simulink model "Simulation"  (R2023a)
settings: Solver=VariableStepAuto  StartTime=0.0  StopTime=5.0  RelTol=1e-3
values from neighbouring files (symbols this model uses):
  Bm = 0.00071*2    (= 0.00142)    [induction_parameter.m]
  J = 0.0038*1.5    (= 0.0057)    [induction_parameter.m]
  Llr = Lls    (= 0.303)    [induction_parameter.m]
  Lls = 4.928-4.625    (= 0.303)    [induction_parameter.m]
  Lm = Lms    (= 4.625)    [induction_parameter.m]
  omega = 0    [induction_parameter.m]
  p = 4    [induction_parameter.m]
  r_r = 40.5    [induction_parameter.m]
  r_s = 79.13    [induction_parameter.m]
  Vm = 310    [induction_parameter.m]
settings Model: Creator=QUDUS  LastModifiedBy=QUDUS

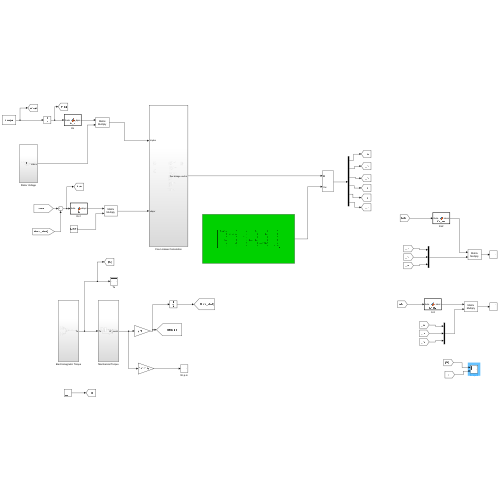
[thumbnail: Simulink's stored preview of the top-level diagram]
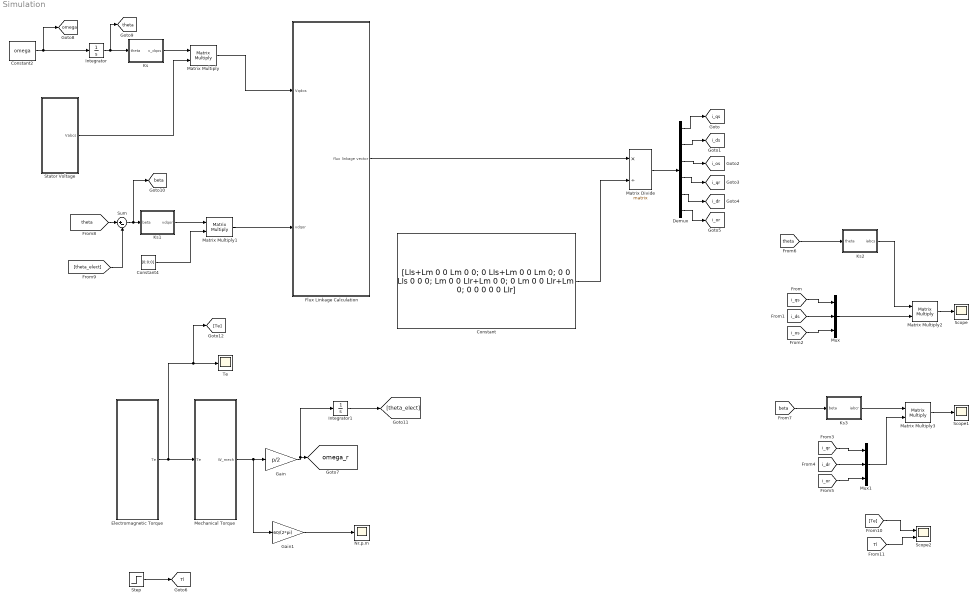
== system Simulation ==
  Constant : Constant  Value=[Lls+Lm 0 0 Lm 0 0; 0 Lls+Lm 0 0 Lm 0; 0 0 Lls 0 0 0; Lm 0 0 Llr+Lm 0 0; 0 Lm 0 0 Llr+Lm 0; 0 0 0 0 0 Llr]
  Constant2 : Constant  Value=omega
  Constant4 : Constant  Value=[0;0;0]
  Demux : Demux  Outputs=6
  Electromagnetic Torque : Subsystem
  Flux Linkage Calculation : Subsystem
  Gain : Gain  Gain=p/2
  Gain1 : Gain  Gain=60/(2*pi)
  Integrator : Integrator
  Integrator1 : Integrator
  Ks : MATLAB Function  TreatAsAtomicUnit=on
  Ks1 : MATLAB Function  TreatAsAtomicUnit=on
  Ks2 : MATLAB Function  TreatAsAtomicUnit=on
  Ks3 : MATLAB Function  TreatAsAtomicUnit=on
  Matrix Divide : Product  Inputs=*/  Multiplication=Matrix(*)
  Matrix Multiply{,1..3} (4 alike) : Product  Multiplication=Matrix(*)
  Mechanical Torque : Subsystem
  Mux : Mux  Inputs=3
  Mux1 : Mux  Inputs=3
  Nr.p.m : Scope
  Scope : Scope
  Scope1 : Scope
  Scope2 : Scope  NumInputPorts=2
  Stator Voltage : Subsystem
  Step : Step  Time=3  After=0.6  SampleTime=0
  Sum : Sum  Inputs=|+-
  Te : Scope
  tag scope: Tl=global, beta=global, i_dr=global, i_ds=global, i_or=global, i_os=global, i_qr=global, i_qs=global, omega=global, omega_r=global, theta=global
  wires:
  Flux Linkage Calculation/1(flux linkage vector) -> Matrix Divide/1
  Constant/1 -> Matrix Divide/2
  Matrix Divide/1 -> Demux/1
  Demux/1 -> [i_qs]
  Demux/2 -> [i_ds]
  Demux/3 -> [i_os]
  Demux/4 -> [i_qr]
  Demux/5 -> [i_dr]
  Demux/6 -> [i_or]
  Step/1 -> [Tl]
  Mechanical Torque/1(W_mech) -> Gain1/1, Gain/1
  Gain1/1 -> Nr.p.m/1
  Gain/1 -> Integrator1/1, [omega_r]
  Ks/1(v_dqos) -> Matrix Multiply/1
  Matrix Multiply/1 -> Flux Linkage Calculation/1(Vqdos)
  Constant2/1 -> Integrator/1, [omega]
  Integrator/1 -> [theta], Ks/1(theta)
  Stator Voltage/1(Vabcs) -> Matrix Multiply/2
  Ks1/1(vdqor) -> Matrix Multiply1/1
  Matrix Multiply1/1 -> Flux Linkage Calculation/2(vdqor)
  Constant4/1 -> Matrix Multiply1/2
  Sum/1 -> [beta], Ks1/1(beta)
  [i_qs] -> Mux/1
  [i_ds] -> Mux/2
  [i_os] -> Mux/3
  Matrix Multiply2/1 -> Scope/1
  [beta] -> Ks3/1(beta)
  Matrix Multiply3/1 -> Scope1/1
  Integrator1/1 -> [theta_elect]
  [theta] -> Sum/1
  [theta_elect] -> Sum/2
  [theta] -> Ks2/1(theta)
  Ks2/1(iabcs) -> Matrix Multiply2/1
  Mux/1 -> Matrix Multiply2/2
  [i_qr] -> Mux1/1
  [i_dr] -> Mux1/2
  [i_or] -> Mux1/3
  Ks3/1(iabcr) -> Matrix Multiply3/1
  Mux1/1 -> Matrix Multiply3/2
  Electromagnetic Torque/1(Te) -> [Te], Te/1, Mechanical Torque/1(Te)
  [Te] -> Scope2/1
  [Tl] -> Scope2/2

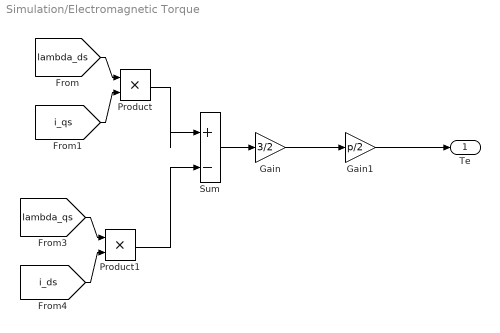
== system Simulation/Electromagnetic Torque ==
  Gain : Gain  Gain=3/2
  Gain1 : Gain  Gain=p/2
  Product : Product
  Product1 : Product
  Sum : Sum  Inputs=|+-
  Te : Outport
  wires:
  Sum/1 -> Gain/1
  Gain/1 -> Gain1/1
  Gain1/1 -> Te/1
  [lambda_ds] -> Product/1
  [i_qs] -> Product/2
  Product/1 -> Sum/1
  [lambda_qs] -> Product1/1
  [i_ds] -> Product1/2
  Product1/1 -> Sum/2

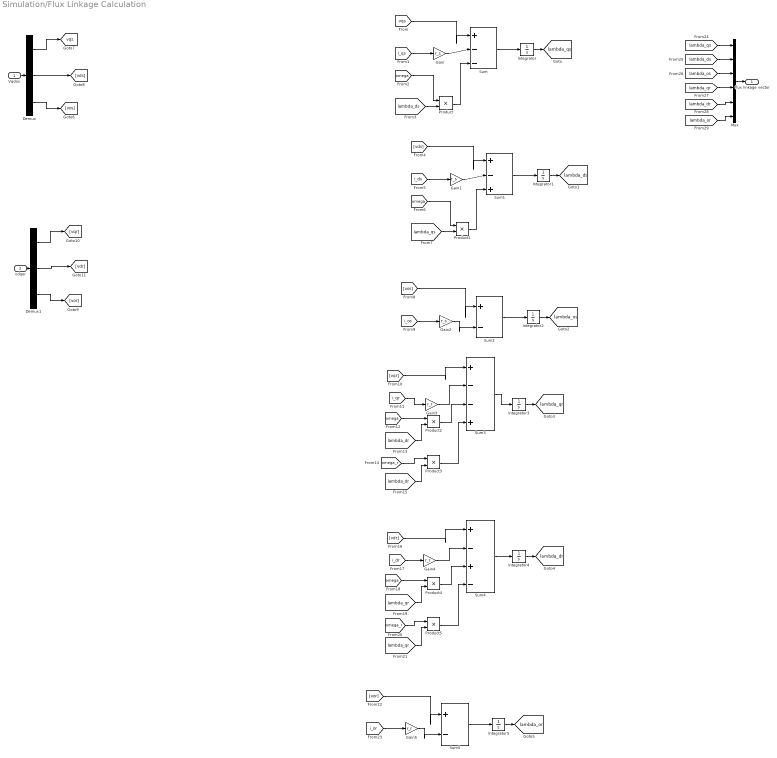
== system Simulation/Flux Linkage Calculation ==
  Vqdos : Inport
  vdqor : Inport  Port=2
  Demux : Demux  Outputs=3
  Demux1 : Demux  Outputs=3
  Gain : Gain  Gain=r_s
  Gain1 : Gain  Gain=r_s
  Gain2 : Gain  Gain=r_s
  Gain3 : Gain  Gain=r_r
  Gain4 : Gain  Gain=r_r
  Gain5 : Gain  Gain=r_r
  Integrator{,1..5} (6 alike) : Integrator
  Mux : Mux  Inputs=6
  Product{,1..5} (6 alike) : Product
  Sum : Sum  Inputs=|+--
  Sum1 : Sum  Inputs=|+-+
  Sum2 : Sum  Inputs=|+-
  Sum3 : Sum  Inputs=|+--+
  Sum4 : Sum  Inputs=|+-+-
  Sum5 : Sum  Inputs=|+-
  flux linkage vector : Outport
  tag scope: lambda_dr=global, lambda_ds=global, lambda_or=global, lambda_os=global, lambda_qr=global, lambda_qs=global, vqs=global
  wires:
  [omega] -> Product/1
  [vqs] -> Sum/1
  [i_qs] -> Gain/1
  Integrator/1 -> [lambda_qs]
  Product/1 -> Sum/3
  Gain/1 -> Sum/2
  [lambda_ds] -> Product/2
  Sum/1 -> Integrator/1
  Sum1/1 -> Integrator1/1
  [lambda_qs] -> Product1/2
  Integrator1/1 -> [lambda_ds]
  Product1/1 -> Sum1/3
  Gain1/1 -> Sum1/2
  [vds] -> Sum1/1
  [omega] -> Product1/1
  [i_ds] -> Gain1/1
  Gain2/1 -> Sum2/2
  Integrator2/1 -> [lambda_os]
  [vos] -> Sum2/1
  [i_os] -> Gain2/1
  Sum2/1 -> Integrator2/1
  Gain3/1 -> Sum3/2
  Integrator3/1 -> [lambda_qr]
  [vqr] -> Sum3/1
  Product2/1 -> Sum3/3
  [i_qr] -> Gain3/1
  [lambda_dr] -> Product2/2
  [omega] -> Product2/1
  Sum3/1 -> Integrator3/1
  [lambda_dr] -> Product3/2
  [omega_r] -> Product3/1
  Product3/1 -> Sum3/4
  Sum4/1 -> Integrator4/1
  [lambda_qr] -> Product4/2
  [i_dr] -> Gain4/1
  [omega] -> Product4/1
  Product4/1 -> Sum4/3
  [lambda_qr] -> Product5/2
  Product5/1 -> Sum4/4
  [omega_r] -> Product5/1
  [vdr] -> Sum4/1
  Integrator4/1 -> [lambda_dr]
  Gain4/1 -> Sum4/2
  [i_or] -> Gain5/1
  Integrator5/1 -> [lambda_or]
  Sum5/1 -> Integrator5/1
  [vor] -> Sum5/1
  Gain5/1 -> Sum5/2
  Demux/3 -> [vos]
  Demux/1 -> [vqs]
  Demux/2 -> [vds]
  Demux1/1 -> [vqr]
  Demux1/2 -> [vdr]
  Demux1/3 -> [vor]
  Vqdos/1 -> Demux/1
  vdqor/1 -> Demux1/1
  [lambda_qs] -> Mux/1
  [lambda_ds] -> Mux/2
  [lambda_os] -> Mux/3
  [lambda_qr] -> Mux/4
  [lambda_dr] -> Mux/5
  [lambda_or] -> Mux/6
  Mux/1 -> flux linkage vector/1

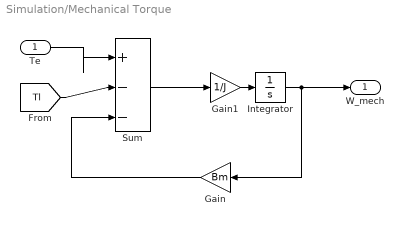
== system Simulation/Mechanical Torque ==
  Te : Inport
  Gain : Gain  Gain=Bm
  Gain1 : Gain  Gain=1/J
  Integrator : Integrator
  Sum : Sum  Inputs=|+--
  W_mech : Outport
  wires:
  Sum/1 -> Gain1/1
  Te/1 -> Sum/1
  [Tl] -> Sum/2
  Gain1/1 -> Integrator/1
  Integrator/1 -> W_mech/1, Gain/1
  Gain/1 -> Sum/3

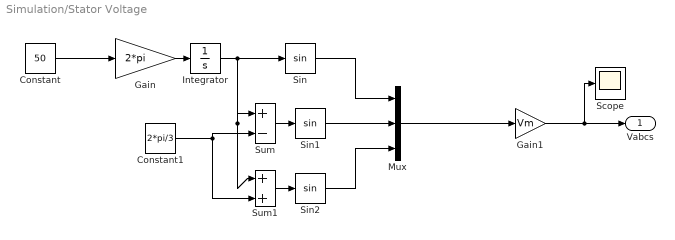
== system Simulation/Stator Voltage ==
  Constant : Constant  Value=50
  Constant1 : Constant  Value=2*pi/3
  Gain : Gain  Gain=2*pi
  Gain1 : Gain  Gain=Vm
  Integrator : Integrator
  Mux : Mux  Inputs=3
  Scope : Scope
  Sin : Trigonometry
  Sin1 : Trigonometry
  Sin2 : Trigonometry
  Sum : Sum  Inputs=|+-
  Sum1 : Sum  Inputs=|++
  Vabcs : Outport
  wires:
  Constant/1 -> Gain/1
  Gain/1 -> Integrator/1
  Integrator/1 -> Sum1/1, Sum/1, Sin/1
  Sin/1 -> Mux/1
  Sin1/1 -> Mux/2
  Sin2/1 -> Mux/3
  Sum/1 -> Sin1/1
  Constant1/1 -> Sum1/2, Sum/2
  Sum1/1 -> Sin2/1
  Mux/1 -> Gain1/1
  Gain1/1 -> Scope/1, Vabcs/1

== matlab function Simulation/Ks ==
  data: theta input; v_dqos output
function v_dqos = K_s(theta)


v_dqos= 2/3* [cos(theta) cos(theta-2*pi/3) cos(theta+2*pi/3); sin(theta) sin(theta-2*pi/3) sin(theta+2*pi/3); 1/2 1/2 1/2];

end

== matlab function Simulation/Ks2 ==
  data: theta input; iabcs output
function iabcs = Ks_inv(theta)


iabcs=[cos(theta) sin(theta) 1; cos(theta-2*pi/3) sin(theta-2*pi/3) 1; cos(theta+2*pi/3) sin(theta+2*pi/3) 1];
end

== matlab function Simulation/Ks3 ==
  data: beta input; iabcr output
function iabcr = Kr_inv(beta)


iabcr= [cos(beta) sin(beta) 1; cos(beta-2*pi/3) sin(beta-2*pi/3) 1; cos(beta+2*pi/3) sin(beta+2*pi/3) 1];

end

== matlab function Simulation/Ks1 ==
  data: beta input; vdqor output
function vdqor = Kr(beta)


vdqor= 2/3* [cos(beta) cos(beta-2*pi/3) cos(beta+2*pi/2); sin(beta) sin(beta-2*pi/3) sin(beta+2*pi/3); 1/2 1/2 1/2];

end
